simulink model "VendingMachine"  (R2020b)
settings: Solver=VariableStepAuto  StartTime=0.0  StopTime=10.0  RelTol=1e-3
settings Model: Creator=sneha  LastModifiedBy=sneha

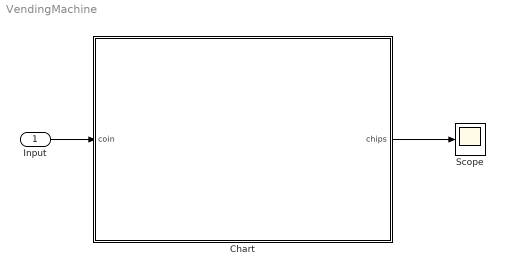
== system VendingMachine ==
  Input : Inport
  Chart : Stateflow chart  TreatAsAtomicUnit=on
  Scope : Scope
  wires:
  Chart/1(chips) -> Scope/1
  Input/1 -> Chart/1(coin)

== stateflow chart VendingMachine/Chart ==
  state GetCoins
  state Coins5
  state Coins10
  (default) -> GetCoins
  GetCoins -> Coins5 [order 1] : [coin==1]{chips=0}
  Coins5 -> GetCoins [order 2] : [coin==2]{chips=1}
  Coins10 -> Coins5 [order 2] : [coin==2]{chips=1}
  GetCoins -> Coins10 [order 2] : [coin==2]{chips=0}
  Coins10 -> GetCoins [order 1] : [coin==1]{chips=1}
  Coins5 -> Coins10 [order 1] : [coin==1]{chips=0}
  data: coin input; chips output
